simulink model "Interpolate"  (R2013b)
settings: Solver=FixedStepDiscrete  StartTime=0.0  StopTime=10  FixedStep=1/800  RelTol=1e-3
InitFcn:
  | s = size(Sad);
  | Time = (0:0.011869:(s(1)-1)*0.011869)';
  | SadTimeSeries = [Time Sad];
  | 
  | s = size(Joy);
  | Time = (0:0.011869:(s(1)-1)*0.011869)';
  | JoyTimeSeries = [Time Joy];
  | 
  | s = size(Anger);
  | Time = (0:0.011869:(s(1)-1)*0.011869)';
  | AngerTimeSeries = [Time Anger];
values from neighbouring files (symbols this model uses):
  Anger = [-2.24 -2.24 -2.24 -2.21 -2.2 -2.22 -2.2 -2.17 -2.15 -2.13 -2.12 -2.09 ... (3206 elements, 3206x1)]    [Emotions_Time_Series.mat]    (also in PNEU_LPF_Analysis.mat)
  Joy = [-1 -1 -1 -1 -0.98 -0.96 -0.86 -0.76 -0.6 -0.46 -0.35 -0.26 ... (2106 elements, 2106x1)]    [Emotions_Time_Series.mat]    (also in PNEU_LPF_Analysis.mat)
  Sad = [4.81 4.88 4.88 4.94 4.94 4.95 4.97 4.93 4.98 4.95 4.95 4.92 ... (3177 elements, 3177x1)]    [Emotions_Time_Series.mat]    (also in PNEU_LPF_Analysis.mat)
undefined symbols (not defined in the file or in its folder): dfilt, fdesignblkfcn, gcbh
libraries: simulink x4, dsparch4 x3
settings Model: Creator=m2memari  LastModifiedBy=m2memari
settings DataIOCC: SignalLoggingSaveFormat=ModelDataLogs
settings DebuggingCC: MultiTaskDSMMsg=warning  MultiTaskCondExecSysMsg=none
settings RTWCC: IncludeERTFirstTime=on

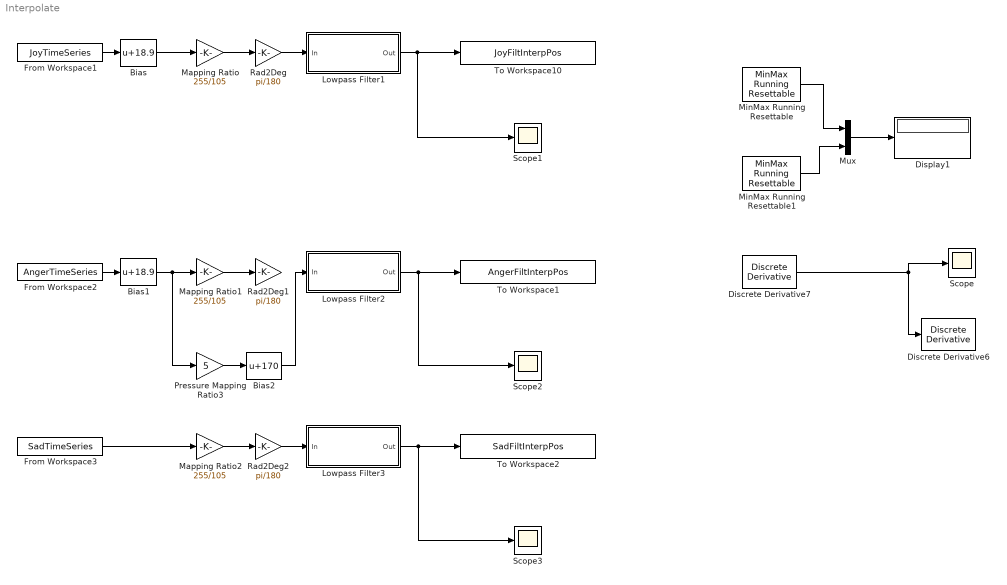
== system Interpolate ==
  Bias : Bias  Bias=18.9
  Bias1 : Bias  Bias=18.9
  Bias2 : Bias  Bias=170
  Discrete Derivative6 : simulink/Discrete/Discrete Derivative  gainval=1.0  ICPrevScaledInput=0.0  InputProcessing=Inherited  OutMin=[]  OutMax=[]  OutDataType=fixdt(1, 16)  OutScaling=2^-10  DoSatur=off
  Discrete Derivative7 : simulink/Discrete/Discrete Derivative  gainval=1.0  ICPrevScaledInput=0.0  InputProcessing=Inherited  OutMin=[]  OutMax=[]  OutDataType=fixdt(1, 16)  OutScaling=2^-10  DoSatur=off
  Display1 : Display
  From Workspace1 : FromWorkspace  VariableName=JoyTimeSeries  SampleTime=1/800  OutputAfterFinalValue=Holding final value
  From Workspace2 : FromWorkspace  VariableName=AngerTimeSeries  SampleTime=1/800  OutputAfterFinalValue=Holding final value
  From Workspace3 : FromWorkspace  VariableName=SadTimeSeries  SampleTime=1/800  OutputAfterFinalValue=Holding final value
  Lowpass Filter1 : Subsystem  DialogController=fdesignblkfcn  InitFcn=fdesignblkfcn(gcbh, {'InitFcn'});  mask(Lowpass Filter){}
      mask help: Design a lowpass filter
      settings: CopyFcn=fdesignblkfcn(gcbh, {'CopyFcn'});
      mask Help: helpview(mapfilelocation('dsp'), 'dsplowpassfilter');
      mask Display: disp('Lowpass')
  Lowpass Filter2 : Subsystem  DialogController=fdesignblkfcn  InitFcn=fdesignblkfcn(gcbh, {'InitFcn'});  mask(Lowpass Filter){}
      mask help: Design a lowpass filter
      settings: CopyFcn=fdesignblkfcn(gcbh, {'CopyFcn'});
      mask Help: helpview(mapfilelocation('dsp'), 'dsplowpassfilter');
      mask Display: disp('Lowpass')
  Lowpass Filter3 : Subsystem  DialogController=fdesignblkfcn  InitFcn=fdesignblkfcn(gcbh, {'InitFcn'});  mask(Lowpass Filter){}
      mask help: Design a lowpass filter
      settings: CopyFcn=fdesignblkfcn(gcbh, {'CopyFcn'});
      mask Help: helpview(mapfilelocation('dsp'), 'dsplowpassfilter');
      mask Display: disp('Lowpass')
  Mapping Ratio : Gain  Gain=255/105
  Mapping Ratio1 : Gain  Gain=255/105
  Mapping Ratio2 : Gain  Gain=255/105
  MinMax Running Resettable : simulink/Math Operations/MinMax Running Resettable  Function=max  vinit=0.0
  MinMax Running Resettable1 : simulink/Math Operations/MinMax Running Resettable  Function=min  vinit=0.0
  Mux : Mux  Inputs=2
  Pressure Mapping Ratio3 : Gain  Gain=5
  Rad2Deg : Gain  Gain=pi/180
  Rad2Deg1 : Gain  Gain=pi/180
  Rad2Deg2 : Gain  Gain=pi/180
  Scope{,1..3} (4 alike) : Scope
      Scope2 settings: SaveName=ScopeData2
      Scope3 settings: SaveName=ScopeData3
  To Workspace1 : ToWorkspace  VariableName=AngerFiltInterpPos  SampleTime=-1  SaveFormat=Timeseries
  To Workspace10 : ToWorkspace  VariableName=JoyFiltInterpPos  SampleTime=-1  SaveFormat=Timeseries
  To Workspace2 : ToWorkspace  VariableName=SadFiltInterpPos  SampleTime=-1  SaveFormat=Timeseries
  wires:
  From Workspace2/1 -> Bias1/1
  MinMax Running Resettable/1 -> Mux/1
  Mapping Ratio/1 -> Rad2Deg/1
  Mapping Ratio1/1 -> Rad2Deg1/1
  MinMax Running Resettable1/1 -> Mux/2
  Mux/1 -> Display1/1
  From Workspace1/1 -> Bias/1
  Discrete Derivative7/1 -> Scope/1, Discrete Derivative6/1
  Lowpass Filter1/1(Out) -> Scope1/1, To Workspace10/1
  Lowpass Filter2/1(Out) -> Scope2/1, To Workspace1/1
  From Workspace3/1 -> Mapping Ratio2/1
  Mapping Ratio2/1 -> Rad2Deg2/1
  Rad2Deg2/1 -> Lowpass Filter3/1(In)
  Lowpass Filter3/1(Out) -> Scope3/1, To Workspace2/1
  Bias/1 -> Mapping Ratio/1
  Bias1/1 -> Pressure Mapping Ratio3/1, Mapping Ratio1/1
  Rad2Deg/1 -> Lowpass Filter1/1(In)
  Pressure Mapping Ratio3/1 -> Bias2/1
  Bias2/1 -> Lowpass Filter2/1(In)

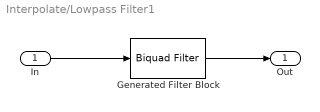
== system Interpolate/Lowpass Filter1 ==
  In : Inport
  Generated Filter Block : dsparch4/Biquad Filter  Tag=BlockMethodSubSystem  IIRFiltStruct=Direct form II  CoeffSource=Specify via dialog  BiQuadCoeffs=[1 2 1 1 -1.5771391443436769 0.96395840320997617;1 2 1 1 -1.5223744078571029 0.89576171631134127;1 2 1 1 -1.4715665227548447 0.83249236353813882;1 2 1 1 -1.4244783961832101 0.77385510112318434;1 2 1 1 -1.3808842706756885 0.719568800876216;1 2 1 1 -1.3405710405656284 0.66936808946838544;1 2 1 1 -1.3033389746124462 0.62300424829440326;1 2 1 1 -1.2690019996571071 0.58024556669918348;1 2 1 1 -1.2373876667761401 0.54087729983057364;1 2 1 1 -1.2083368942636938 0.50470134858354321;1 2 1 1 -1.1817035599733907 0.47153575195718578;1 2 1 1 -1.1573539982383976 0.44121406058618068;1 2 1 1 -1.1351664429699106 0.4135846432500429;1 2 1 1 -1.1150304479172246 0.38850996494245799;1 2 1 1 -1.0968463068653984 0.36586586486291095;1 2 1 1 -1.0805244902565045 0.34554085486004982;1 2 1 1 -1.065985109943663 0.32743545290786247;1 2 1 1 -1.053157420196817 0.31146156172493034;1 2 1 1 -1.041979360413757 0.29754189932782449;1 2 1 1 -1.032397143041319 0.28560948588321666;1 2 1 1 -1.0243648888158372 0.2756071894850643;1 2 1 1 -1.0178443104598014 0.26748733227268423;1 2 1 1 -1.0128044453223521 0.26121135749694074;1 2 1 1 -1.0092214370457362 0.25674955763681551;1 2 1 1 -1.0070783661163576 0.25408086339032315;1 1 0 1 -0.50318256453445276 0]  a0Flag=Warning  IC=0  ICnum=0  ICden=0  InputProcessing=Columns as channels (frame based)  denAccumFracLength=30  denProdOutputFracLength=30  secondMemoryFracLength=15  roundingMode=Floor  overflowMode=off  ScaleValues=[0.096704814716574869;0.093346827113559599;0.09023146019582351;0.087344176234993562;0.084671132550131908;0.082199262225689254;0.079916318420489282;0.077810891760519113;0.075872408263608429;0.07409111357996237;0.072458047995948752;0.07096501558694579;0.069604550070033064;0.068369879256308372;0.067254889499378148;0.066254091150886305;0.065362585741049875;0.064576035382028343;0.063890634728516901;0.063303085710474383;0.062810575167306745;0.062410755453220723;0.062101728043647185;0.061882030147769843;0.061750624318491369;0.24840871773277368;1]  optimizeScaleValues=off  ScaleValueMode=Specify via input port (g)  scaleValueFracLength=14  FilterSource=Specify via dialog  dfiltObjectName=dfilt.df2tsos([1 0.3 0.4],[1 0.1 0.2])
  Out : Outport
  wires:
  Generated Filter Block/1 -> Out/1
  In/1 -> Generated Filter Block/1

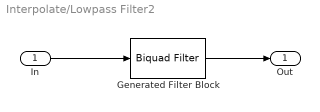
== system Interpolate/Lowpass Filter2 ==
  In : Inport
  Generated Filter Block : dsparch4/Biquad Filter  Tag=BlockMethodSubSystem  IIRFiltStruct=Direct form II  CoeffSource=Specify via dialog  BiQuadCoeffs=[1 2 1 1 -1.5771391443436769 0.96395840320997617;1 2 1 1 -1.5223744078571029 0.89576171631134127;1 2 1 1 -1.4715665227548447 0.83249236353813882;1 2 1 1 -1.4244783961832101 0.77385510112318434;1 2 1 1 -1.3808842706756885 0.719568800876216;1 2 1 1 -1.3405710405656284 0.66936808946838544;1 2 1 1 -1.3033389746124462 0.62300424829440326;1 2 1 1 -1.2690019996571071 0.58024556669918348;1 2 1 1 -1.2373876667761401 0.54087729983057364;1 2 1 1 -1.2083368942636938 0.50470134858354321;1 2 1 1 -1.1817035599733907 0.47153575195718578;1 2 1 1 -1.1573539982383976 0.44121406058618068;1 2 1 1 -1.1351664429699106 0.4135846432500429;1 2 1 1 -1.1150304479172246 0.38850996494245799;1 2 1 1 -1.0968463068653984 0.36586586486291095;1 2 1 1 -1.0805244902565045 0.34554085486004982;1 2 1 1 -1.065985109943663 0.32743545290786247;1 2 1 1 -1.053157420196817 0.31146156172493034;1 2 1 1 -1.041979360413757 0.29754189932782449;1 2 1 1 -1.032397143041319 0.28560948588321666;1 2 1 1 -1.0243648888158372 0.2756071894850643;1 2 1 1 -1.0178443104598014 0.26748733227268423;1 2 1 1 -1.0128044453223521 0.26121135749694074;1 2 1 1 -1.0092214370457362 0.25674955763681551;1 2 1 1 -1.0070783661163576 0.25408086339032315;1 1 0 1 -0.50318256453445276 0]  a0Flag=Warning  IC=0  ICnum=0  ICden=0  InputProcessing=Columns as channels (frame based)  denAccumFracLength=30  denProdOutputFracLength=30  secondMemoryFracLength=15  roundingMode=Floor  overflowMode=off  ScaleValues=[0.096704814716574869;0.093346827113559599;0.09023146019582351;0.087344176234993562;0.084671132550131908;0.082199262225689254;0.079916318420489282;0.077810891760519113;0.075872408263608429;0.07409111357996237;0.072458047995948752;0.07096501558694579;0.069604550070033064;0.068369879256308372;0.067254889499378148;0.066254091150886305;0.065362585741049875;0.064576035382028343;0.063890634728516901;0.063303085710474383;0.062810575167306745;0.062410755453220723;0.062101728043647185;0.061882030147769843;0.061750624318491369;0.24840871773277368;1]  optimizeScaleValues=off  ScaleValueMode=Specify via input port (g)  scaleValueFracLength=14  FilterSource=Specify via dialog  dfiltObjectName=dfilt.df2tsos([1 0.3 0.4],[1 0.1 0.2])
  Out : Outport
  wires:
  In/1 -> Generated Filter Block/1
  Generated Filter Block/1 -> Out/1

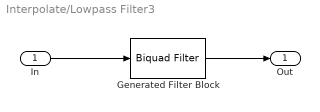
== system Interpolate/Lowpass Filter3 ==
  In : Inport
  Generated Filter Block : dsparch4/Biquad Filter  Tag=BlockMethodSubSystem  IIRFiltStruct=Direct form II  CoeffSource=Specify via dialog  BiQuadCoeffs=[1 2 1 1 -1.5771391443436769 0.96395840320997617;1 2 1 1 -1.5223744078571029 0.89576171631134127;1 2 1 1 -1.4715665227548447 0.83249236353813882;1 2 1 1 -1.4244783961832101 0.77385510112318434;1 2 1 1 -1.3808842706756885 0.719568800876216;1 2 1 1 -1.3405710405656284 0.66936808946838544;1 2 1 1 -1.3033389746124462 0.62300424829440326;1 2 1 1 -1.2690019996571071 0.58024556669918348;1 2 1 1 -1.2373876667761401 0.54087729983057364;1 2 1 1 -1.2083368942636938 0.50470134858354321;1 2 1 1 -1.1817035599733907 0.47153575195718578;1 2 1 1 -1.1573539982383976 0.44121406058618068;1 2 1 1 -1.1351664429699106 0.4135846432500429;1 2 1 1 -1.1150304479172246 0.38850996494245799;1 2 1 1 -1.0968463068653984 0.36586586486291095;1 2 1 1 -1.0805244902565045 0.34554085486004982;1 2 1 1 -1.065985109943663 0.32743545290786247;1 2 1 1 -1.053157420196817 0.31146156172493034;1 2 1 1 -1.041979360413757 0.29754189932782449;1 2 1 1 -1.032397143041319 0.28560948588321666;1 2 1 1 -1.0243648888158372 0.2756071894850643;1 2 1 1 -1.0178443104598014 0.26748733227268423;1 2 1 1 -1.0128044453223521 0.26121135749694074;1 2 1 1 -1.0092214370457362 0.25674955763681551;1 2 1 1 -1.0070783661163576 0.25408086339032315;1 1 0 1 -0.50318256453445276 0]  a0Flag=Warning  IC=0  ICnum=0  ICden=0  InputProcessing=Columns as channels (frame based)  denAccumFracLength=30  denProdOutputFracLength=30  secondMemoryFracLength=15  roundingMode=Floor  overflowMode=off  ScaleValues=[0.096704814716574869;0.093346827113559599;0.09023146019582351;0.087344176234993562;0.084671132550131908;0.082199262225689254;0.079916318420489282;0.077810891760519113;0.075872408263608429;0.07409111357996237;0.072458047995948752;0.07096501558694579;0.069604550070033064;0.068369879256308372;0.067254889499378148;0.066254091150886305;0.065362585741049875;0.064576035382028343;0.063890634728516901;0.063303085710474383;0.062810575167306745;0.062410755453220723;0.062101728043647185;0.061882030147769843;0.061750624318491369;0.24840871773277368;1]  optimizeScaleValues=off  ScaleValueMode=Specify via input port (g)  scaleValueFracLength=14  FilterSource=Specify via dialog  dfiltObjectName=dfilt.df2tsos([1 0.3 0.4],[1 0.1 0.2])
  Out : Outport
  wires:
  Generated Filter Block/1 -> Out/1
  In/1 -> Generated Filter Block/1
